simulink model "course_loop"  (R2014b)
settings: Solver=ode45  StartTime=0.0  StopTime=10.0  MaxStep=0.1  RelTol=1e-3
values from neighbouring files (symbols this model uses):
  a_phi_1 = -(1/2)*P.rho * Va^2 * P.S_wing * P.b * P.C_p_p * P.b / (2*Va)    [roll_hold_tuning.m]
  a_phi_2 = (1/2)*P.rho * Va^2 * P.S_wing * P.b * P.C_p_delta_a    [roll_hold_tuning.m]
  k_d_phi = (2*zeta_phi*w_n_phi - a_phi_1)/a_phi_2    [roll_hold_tuning.m]
  k_i_phi = 1.05    [roll_hold_tuning.m]
  k_p_phi = delta_a_max/e_phi_max * sign(a_phi_2)    [roll_hold_tuning.m]
undefined symbols (not defined in the file or in its folder): k_i_chi, k_p_chi, P, Vg
settings Model: Creator=kunalmenda  LastModifiedBy=kunalmenda

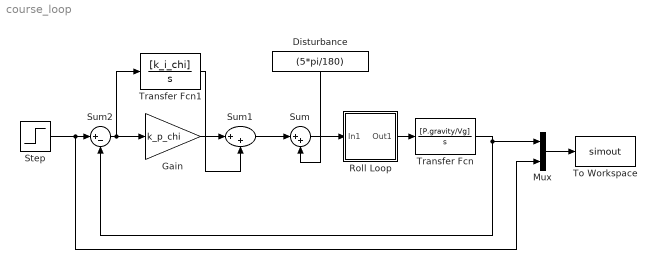
== system course_loop ==
  Disturbance : Constant  Value=(5*pi/180)
  Gain : Gain  Gain=k_p_chi
  Mux : Mux  Inputs=2
  "Roll Loop " : Subsystem
  Step : Step  After=25*pi/180  SampleTime=0
  Sum : Sum  Inputs=|++
  Sum1 : Sum  Inputs=|++
  Sum2 : Sum  Inputs=|+-
  To Workspace : ToWorkspace  VariableName=simout  SaveFormat=Timeseries  SampleTime=-1
  Transfer Fcn : TransferFcn  Numerator=[P.gravity/Vg]  Denominator=[1 0]
  Transfer Fcn1 : TransferFcn  Numerator=[k_i_chi]  Denominator=[1 0]
  wires:
  Sum2/1 -> Transfer Fcn1/1, Gain/1
  Disturbance/1 -> Sum/2
  Transfer Fcn/1 -> Mux/1, Sum2/2
  Step/1 -> Mux/2, Sum2/1
  Mux/1 -> To Workspace/1
  Sum1/1 -> Sum/1
  Gain/1 -> Sum1/1
  Transfer Fcn1/1 -> Sum1/2
  "Roll Loop "/1(Out1) -> Transfer Fcn/1
  Sum/1 -> "Roll Loop "/1(In1)

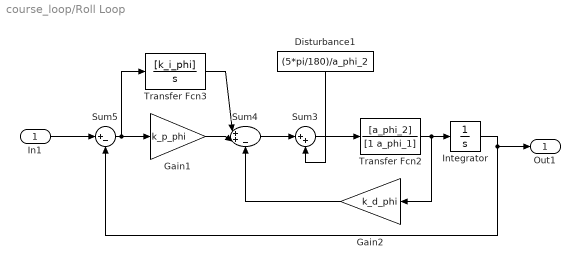
== system course_loop/Roll Loop  ==
  In1 : Inport
  Disturbance1 : Constant  Value=(5*pi/180)/a_phi_2
  Gain1 : Gain  Gain=k_p_phi
  Gain2 : Gain  Gain=k_d_phi
  Integrator : Integrator
  Sum3 : Sum  Inputs=|++
  Sum4 : Sum  Inputs=|++-
  Sum5 : Sum  Inputs=|+-
  Transfer Fcn2 : TransferFcn  Numerator=[a_phi_2]  Denominator=[1 a_phi_1]
  Transfer Fcn3 : TransferFcn  Numerator=[k_i_phi]  Denominator=[1 0]
  Out1 : Outport
  wires:
  Sum5/1 -> Transfer Fcn3/1, Gain1/1
  Transfer Fcn2/1 -> Gain2/1, Integrator/1
  Integrator/1 -> Out1/1, Sum5/2
  Transfer Fcn3/1 -> Sum4/1
  Gain2/1 -> Sum4/3
  Sum4/1 -> Sum3/1
  Disturbance1/1 -> Sum3/2
  In1/1 -> Sum5/1
  Gain1/1 -> Sum4/2
  Sum3/1 -> Transfer Fcn2/1
